simulink model "linearspring"  (Simulink 7.8)
settings: Solver=ode1  StartTime=0.0  StopTime=100.0  FixedStep=0.01  RelTol=1e-3
settings Model: Creator=stepp  LastModifiedBy=stepp
settings DataIOCC: LimitDataPoints=off  SaveOutput=off  SaveState=on  StateSaveName=x  TimeSaveName=t

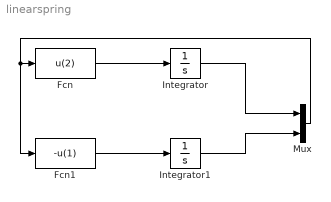
== system linearspring ==
  Fcn : Fcn  Expr=u(2)
  Fcn1 : Fcn  Expr=-u(1)
  Integrator : Integrator
  Integrator1 : Integrator  InitialCondition=1
  Mux : Mux  Inputs=2
  wires:
  Fcn/1 -> Integrator/1
  Fcn1/1 -> Integrator1/1
  Integrator/1 -> Mux/1
  Integrator1/1 -> Mux/2
  Mux/1 -> Fcn/1, Fcn1/1
